simulink model "TorqueControl_QuadRad_MPC"  (R2015b)
settings: Solver=ode4  StartTime=0.0  StopTime=2000  FixedStep=1  RelTol=1e-3
values from neighbouring files (symbols this model uses):
  bicycle = initBicycle(60, 0.01468, 0.79, 0.33, 0.17, 5.5, 24, 50, 48)    [RunSimulinkSim_MPC.m]
  cyclist = initCyclist(0, 30, 183, 75, 80)    [RunSimulinkSim_MPC.m]
  environment = initEnvironment_V2(altitude, distance, fRES, 9.81, 1.2041)    [RunSimulinkSim_MPC.m]
  P_M = P_M_ref+fac.*P_M_ref_exc    [RunSimulinkSim_MPC.m]
  system = initHRmodel(0.0113, 0.0072, 0.0049, 0.0041, 19.8002, 0.0072, cyclist.P_max, cyclist.cadence)    [RunSimulinkSim_MPC.m]
undefined symbols (not defined in the file or in its folder): init, mpc, variation
libraries: simulink x2
settings Model: Creator=Daniel  LastModifiedBy=David
settings DataIOCC: SaveFormat=Array

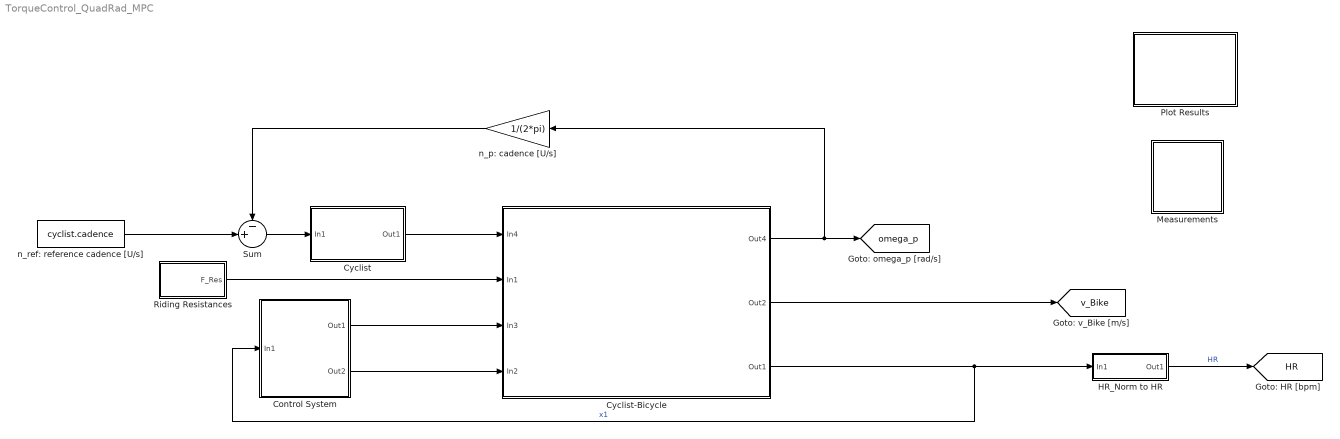
== system TorqueControl_QuadRad_MPC ==
  Control System : Subsystem
  Cyclist : Subsystem
  Cyclist-Bicycle : Subsystem
  HR_Norm to HR : Subsystem
  Measurements : Subsystem
  Plot Results : Subsystem
  Riding Resistances : Subsystem
  Sum : Sum  Inputs=-+|
  n_p: cadence [U/s] : Gain  Gain=1/(2*pi)
  n_ref: reference cadence [U/s] : Constant  Value=cyclist.cadence
  tag scope: HR=global, omega_p=global, v_Bike=global
  wires:
  Cyclist-Bicycle/1(Out4) -> n_p: cadence [U/s]/1, [omega_p]
  n_ref: reference cadence [U/s]/1 -> Sum/2
  n_p: cadence [U/s]/1 -> Sum/1
  Riding Resistances/1(F_Res) -> Cyclist-Bicycle/2(In1)
  Cyclist-Bicycle/2(Out2) -> [v_Bike]
  Cyclist-Bicycle/3(Out1) -> Control System/1(In1), HR_Norm to HR/1(In1)  "x1"
  HR_Norm to HR/1(Out1) -> [HR]  "HR"
  Sum/1 -> Cyclist/1(In1)
  Cyclist/1(Out1) -> Cyclist-Bicycle/1(In4)
  Control System/1(Out1) -> Cyclist-Bicycle/3(In3)
  Control System/2(Out2) -> Cyclist-Bicycle/4(In2)

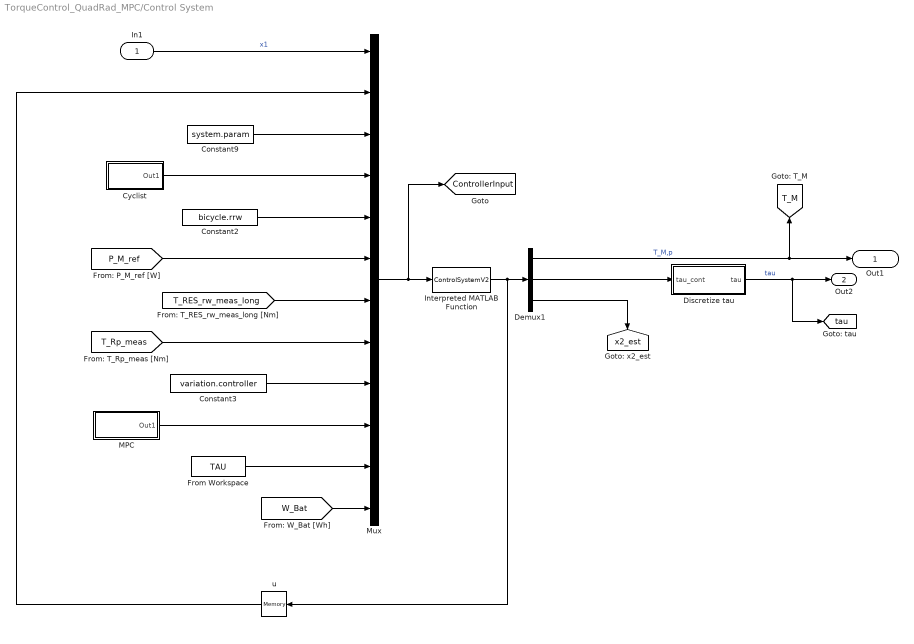
== system TorqueControl_QuadRad_MPC/Control System ==
  In1 : Inport
  Constant2 : Constant  Value=bicycle.rrw
  Constant3 : Constant  Value=variation.controller
  Constant9 : Constant  Value=system.param
  Cyclist : Subsystem
  Demux1 : Demux  Outputs=3
  Discretize tau : MATLAB Function  TreatAsAtomicUnit=on
  From Workspace : FromWorkspace  VariableName=TAU  SampleTime=0
  Interpreted MATLAB Function : MATLABFcn  MATLABFcn=ControlSystemV2  OutputDimensions=3
  MPC : Subsystem
  Mux : Mux  Inputs=12
  u : Memory  X0=[0 init.tau init.x2_est]  InheritSampleTime=on
  Out1 : Outport
  Out2 : Outport  Port=2
  tag scope: ControllerInput=global, T_M=global, tau=global, x2_est=global
  wires:
  In1/1 -> Mux/1  "x1"
  Demux1/3 -> [x2_est]
  Constant2/1 -> Mux/5
  Mux/1 -> [ControllerInput], Interpreted MATLAB Function/1
  Interpreted MATLAB Function/1 -> Demux1/1, u/1
  Constant9/1 -> Mux/3
  [T_RES_rw_meas_long] -> Mux/7
  u/1 -> Mux/2
  [P_M_ref] -> Mux/6
  Demux1/1 -> [T_M], Out1/1  "T_M,p"
  Demux1/2 -> Discretize tau/1(tau_cont)
  Discretize tau/1(tau) -> [tau], Out2/1  "tau"
  Cyclist/1(Out1) -> Mux/4
  [T_Rp_meas] -> Mux/8
  From Workspace/1 -> Mux/11
  Constant3/1 -> Mux/9
  MPC/1(Out1) -> Mux/10
  [W_Bat] -> Mux/12

== system TorqueControl_QuadRad_MPC/Cyclist ==
  In1 : Inport
  T_R,p: Rider torque at pedals [Nm] : simulink/Continuous/PID Controller  Controller=PID  TimeDomain=Discrete-time  SampleTime=-1  IntegratorMethod=Forward Euler  FilterMethod=Forward Euler  Form=Parallel  UseFilter=on  ControllerParametersSource=internal  P=300  I=25  D=0  N=1  InitialConditionSource=internal  InitialConditionForIntegrator=0  InitialConditionForFilter=0  ExternalReset=none  LimitOutput=on  UpperSaturationLimit=1000  LowerSaturationLimit=1  LinearizeAsGain=on  AntiWindupMode=none  Kb=1  TrackingMode=off  Kt=1  PParamMin=[]  PParamMax=[]  IParamMin=[]  IParamMax=[]  DParamMin=[]  DParamMax=[]  NParamMin=[]  NParamMax=[]  KbParamMin=[]  KbParamMax=[]  KtParamMin=[]  KtParamMax=[]  POutMin=[]  POutMax=[]  IOutMin=[]  IOutMax=[]  DOutMin=[]  DOutMax=[]  NOutMin=[]  NOutMax=[]  KbOutMin=[]  KbOutMax=[]  KtOutMin=[]  KtOutMax=[]  IntegratorOutMin=[]  IntegratorOutMax=[]  FilterOutMin=[]  FilterOutMax=[]  SumOutMin=[]  SumOutMax=[]  SumI1OutMin=[]  SumI1OutMax=[]  SumI2OutMin=[]  SumI2OutMax=[]  SumI3OutMin=[]  SumI3OutMax=[]  SumDOutMin=[]  SumDOutMax=[]  SaturationOutMin=[]  SaturationOutMax=[]  IntegratorContinuousStateAttributes=''  IntegratorStateMustResolveToSignalObject=off  IntegratorRTWStateStorageClass=Auto  FilterContinuousStateAttributes=''  FilterStateMustResolveToSignalObject=off  FilterRTWStateStorageClass=Auto  DifferentiatorICPrevScaledInput=0  DifferentiatorOutMin=[]  DifferentiatorOutMax=[]
  Out1 : Outport
  tag scope: T_Rp=global
  wires:
  In1/1 -> T_R,p: Rider torque at pedals [Nm]/1  "e_n"
  T_R,p: Rider torque at pedals [Nm]/1 -> [T_Rp], Out1/1  "T_R,p [Nm]"

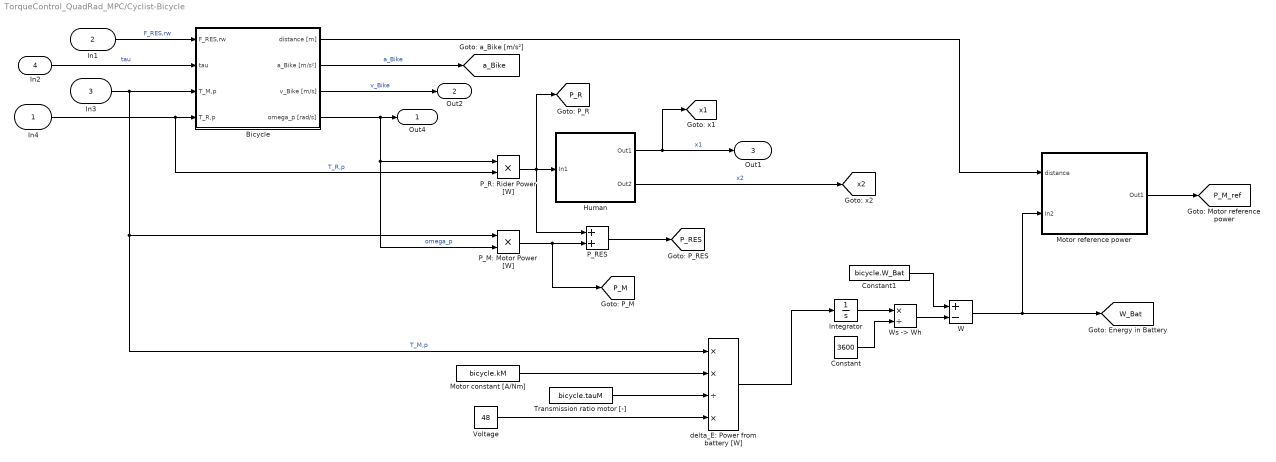
== system TorqueControl_QuadRad_MPC/Cyclist-Bicycle ==
  In4 : Inport
  In1 : Inport  Port=2
  In3 : Inport  Port=3
  In2 : Inport  Port=4
  Bicycle : Subsystem
  Constant : Constant  Value=3600
  Constant1 : Constant  Value=bicycle.W_Bat
  Human : Subsystem
  Integrator : Integrator
  Motor constant [A/Nm] : Constant  Value=bicycle.kM
  Motor reference power : Subsystem
  P_M: Motor Power [W] : Product
  P_R: Rider Power [W] : Product
  P_RES : Sum
  Transmission ratio motor [-] : Constant  Value=bicycle.tauM
  Voltage : Constant  Value=48
  W : Sum  Inputs=+-
  "Ws -> Wh" : Product  Inputs=*/
  delta_E: Power from battery [W] : Product  Inputs=**/*
  Out4 : Outport
  Out2 : Outport  Port=2
  Out1 : Outport  Port=3
  tag scope: P_M=global, P_M_ref=global, P_R=global, P_RES=global, W_Bat=global, a_Bike=global, x1=global, x2=global
  wires:
  P_R: Rider Power [W]/1 -> [P_R], P_RES/1, Human/1(In1)
  Bicycle/3(v_Bike [m/s]) -> Out2/1  "v_Bike"
  Bicycle/2(a_Bike [m/s²]) -> [a_Bike]  "a_Bike"
  Human/2(Out2) -> [x2]  "x2"
  In2/1 -> Bicycle/2(tau)  "tau"
  In3/1 -> P_M: Motor Power [W]/1, delta_E: Power from battery [W]/1, Bicycle/3(T_M,p)  "T_M,p"
  In4/1 -> P_R: Rider Power [W]/2, Bicycle/4(T_R,p)  "T_R,p"
  In1/1 -> Bicycle/1(F_RES,rw)  "F_RES,rw"
  Bicycle/4(omega_p [rad/s]) -> Out4/1, P_M: Motor Power [W]/2, P_R: Rider Power [W]/1  "omega_p"
  Human/1(Out1) -> Out1/1, [x1]  "x1"
  P_M: Motor Power [W]/1 -> [P_M], P_RES/2
  P_RES/1 -> [P_RES]
  Motor constant [A/Nm]/1 -> delta_E: Power from battery [W]/2
  Transmission ratio motor [-]/1 -> delta_E: Power from battery [W]/3
  Voltage/1 -> delta_E: Power from battery [W]/4
  delta_E: Power from battery [W]/1 -> Integrator/1
  Integrator/1 -> "Ws -> Wh"/1
  Constant/1 -> "Ws -> Wh"/2
  "Ws -> Wh"/1 -> W/2
  Constant1/1 -> W/1
  W/1 -> Motor reference power/2(In2), [W_Bat]
  Bicycle/1(distance [m]) -> Motor reference power/1(distance)
  Motor reference power/1(Out1) -> [P_M_ref]

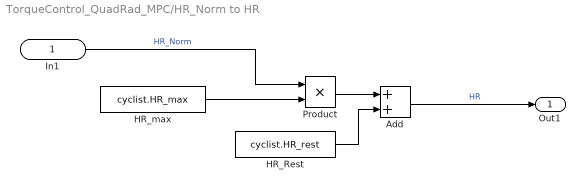
== system TorqueControl_QuadRad_MPC/HR_Norm to HR ==
  In1 : Inport
  Add : Sum
  HR_Rest : Constant  Value=cyclist.HR_rest
  HR_max : Constant  Value=cyclist.HR_max
  Product : Product
  Out1 : Outport
  wires:
  HR_max/1 -> Product/2
  Add/1 -> Out1/1  "HR"
  Product/1 -> Add/1
  HR_Rest/1 -> Add/2
  In1/1 -> Product/1  "HR_Norm"

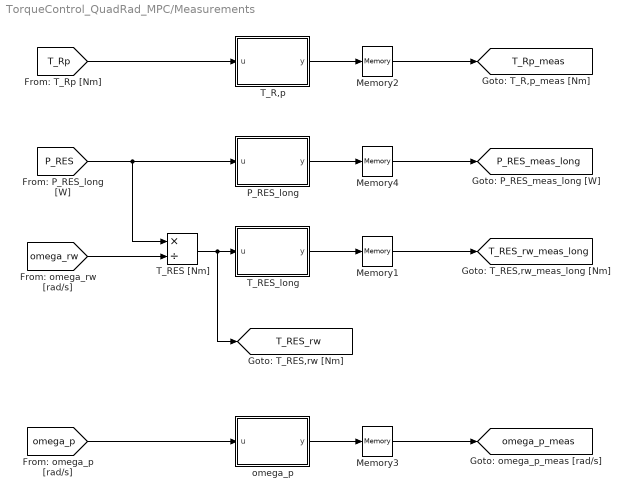
== system TorqueControl_QuadRad_MPC/Measurements ==
  Memory1 : Memory  InheritSampleTime=on
  Memory2 : Memory  InheritSampleTime=on
  Memory3 : Memory  InheritSampleTime=on
  Memory4 : Memory  X0=init.P_RES  InheritSampleTime=on
  P_RES_long : MATLAB Function  TreatAsAtomicUnit=on
  T_R,p : MATLAB Function  TreatAsAtomicUnit=on
  T_RES [Nm] : Product  Inputs=*/
  T_RES_long : MATLAB Function  TreatAsAtomicUnit=on
  omega_p : MATLAB Function  TreatAsAtomicUnit=on
  tag scope: P_RES_meas_long=global, T_RES_rw=global, T_RES_rw_meas_long=global, T_Rp_meas=global, omega_p_meas=global
  wires:
  [P_RES] -> T_RES [Nm]/1, P_RES_long/1(u)
  Memory4/1 -> [P_RES_meas_long]
  P_RES_long/1(y) -> Memory4/1
  [omega_rw] -> T_RES [Nm]/2
  T_RES [Nm]/1 -> [T_RES_rw], T_RES_long/1(u)
  T_RES_long/1(y) -> Memory1/1
  Memory1/1 -> [T_RES_rw_meas_long]
  [T_Rp] -> T_R,p/1(u)
  T_R,p/1(y) -> Memory2/1
  Memory2/1 -> [T_Rp_meas]
  [omega_p] -> omega_p/1(u)
  omega_p/1(y) -> Memory3/1
  Memory3/1 -> [omega_p_meas]

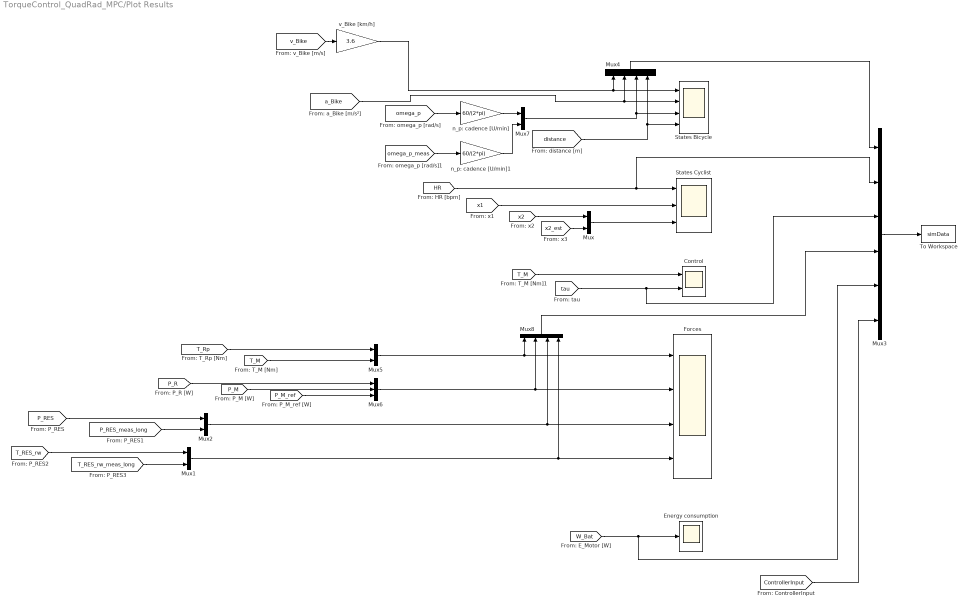
== system TorqueControl_QuadRad_MPC/Plot Results ==
  Control : Scope  NumInputPorts=2
  Energy consumption : Scope
  Forces : Scope  NumInputPorts=4
  Mux{,1..2,5,7} (5 alike) : Mux  Inputs=2
  Mux3 : Mux  Inputs=6
  Mux4 : Mux
  Mux6 : Mux  Inputs=3
  Mux8 : Mux
  States Bicycle : Scope  NumInputPorts=4
  States Cyclist : Scope  NumInputPorts=3
  To Workspace : ToWorkspace  VariableName=simData  SaveFormat=Timeseries  SampleTime=-1
  n_p: cadence [U/min] : Gain  Gain=60/(2*pi)
  n_p: cadence [U/min]1 : Gain  Gain=60/(2*pi)
  v_Bike [km/h] : Gain  Gain=3.6
  wires:
  [omega_p] -> n_p: cadence [U/min]/1
  [v_Bike] -> v_Bike [km/h]/1
  [HR] -> Mux3/2, States Cyclist/1
  [x1] -> States Cyclist/2
  [x2] -> Mux/1
  [P_M] -> Mux6/2
  [P_RES] -> Mux2/1
  [x2_est] -> Mux/2
  Mux/1 -> States Cyclist/3
  [tau] -> Mux3/3, Control/2
  [P_RES_meas_long] -> Mux2/2
  [a_Bike] -> Mux4/2, States Bicycle/2
  [T_Rp] -> Mux5/1
  [P_R] -> Mux6/1
  [distance] -> States Bicycle/4, Mux4/4
  Mux5/1 -> Mux8/1, Forces/1
  Mux6/1 -> Forces/2, Mux8/2
  [T_M] -> Mux5/2
  [T_M] -> Control/1
  Mux2/1 -> Mux8/3, Forces/3
  [T_RES_rw] -> Mux1/1
  [T_RES_rw_meas_long] -> Mux1/2
  Mux1/1 -> Forces/4, Mux8/4
  [P_M_ref] -> Mux6/3
  [W_Bat] -> Mux3/5, Energy consumption/1
  v_Bike [km/h]/1 -> Mux4/1, States Bicycle/1
  Mux3/1 -> To Workspace/1
  Mux4/1 -> Mux3/1
  Mux8/1 -> Mux3/4
  [ControllerInput] -> Mux3/6
  [omega_p_meas] -> n_p: cadence [U/min]1/1
  n_p: cadence [U/min]/1 -> Mux7/1
  n_p: cadence [U/min]1/1 -> Mux7/2
  Mux7/1 -> States Bicycle/3, Mux4/3

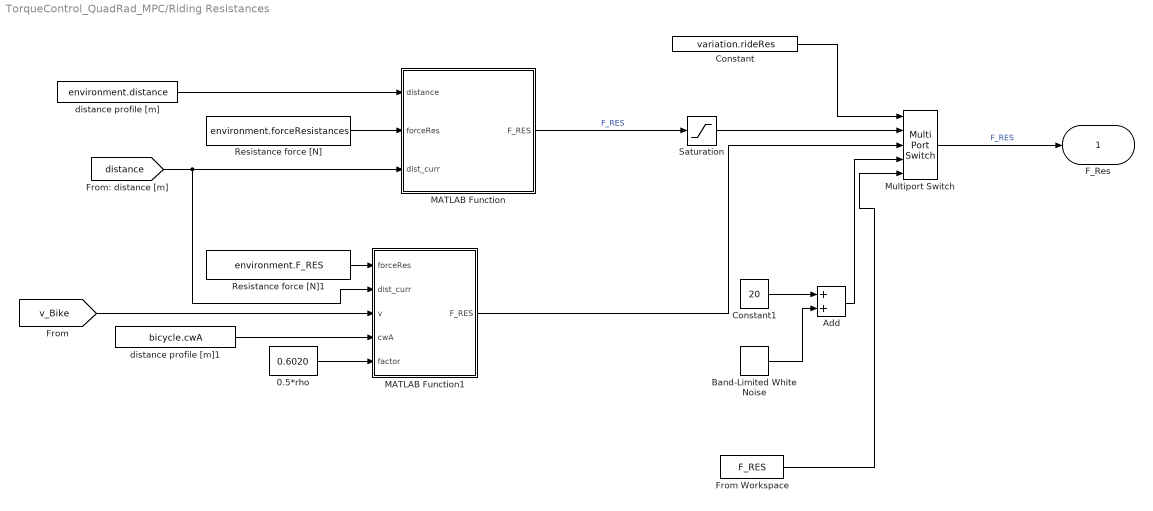
== system TorqueControl_QuadRad_MPC/Riding Resistances ==
  0.5*rho : Constant  Value=0.6020
  Add : Sum
  Band-Limited White Noise : simulink/Sources/Band-Limited White Noise  Cov=[10]  Ts=1  seed=[23341]
  Constant : Constant  Value=variation.rideRes
  Constant1 : Constant  Value=20
  From Workspace : FromWorkspace  VariableName=F_RES  SampleTime=0
  MATLAB Function : MATLAB Function  TreatAsAtomicUnit=on
  MATLAB Function1 : MATLAB Function  TreatAsAtomicUnit=on
  Multiport Switch : MultiPortSwitch  Inputs=4
  Resistance force [N] : Constant  Value=environment.forceResistances
  Resistance force [N]1 : Constant  Value=environment.F_RES
  Saturation : Saturate  UpperLimit=150  LowerLimit=0
  distance profile [m] : Constant  Value=environment.distance
  distance profile [m]1 : Constant  Value=bicycle.cwA
  F_Res : Outport
  wires:
  [distance] -> MATLAB Function/3(dist_curr), MATLAB Function1/2(dist_curr)
  Multiport Switch/1 -> F_Res/1  "F_RES"
  distance profile [m]/1 -> MATLAB Function/1(distance)
  Resistance force [N]/1 -> MATLAB Function/2(forceRes)
  Constant/1 -> Multiport Switch/1
  MATLAB Function/1(F_RES) -> Saturation/1  "F_RES"
  Constant1/1 -> Add/1
  Band-Limited White Noise/1 -> Add/2
  Add/1 -> Multiport Switch/4
  From Workspace/1 -> Multiport Switch/5
  Saturation/1 -> Multiport Switch/2
  [v_Bike] -> MATLAB Function1/3(v)
  distance profile [m]1/1 -> MATLAB Function1/4(cwA)
  0.5*rho/1 -> MATLAB Function1/5(factor)
  Resistance force [N]1/1 -> MATLAB Function1/1(forceRes)
  MATLAB Function1/1(F_RES) -> Multiport Switch/3

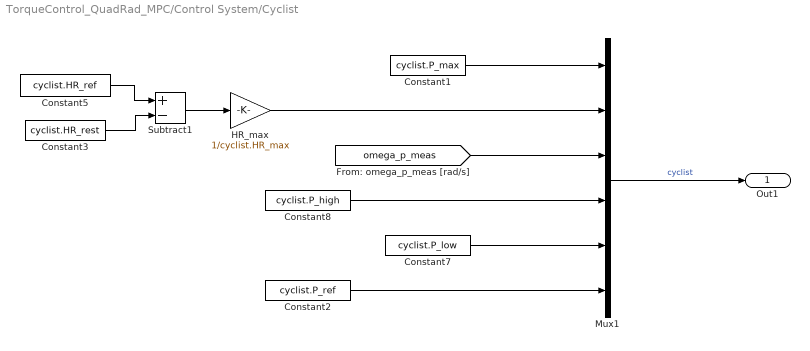
== system TorqueControl_QuadRad_MPC/Control System/Cyclist ==
  Constant1 : Constant  Value=cyclist.P_max
  Constant2 : Constant  Value=cyclist.P_ref
  Constant3 : Constant  Value=cyclist.HR_rest
  Constant5 : Constant  Value=cyclist.HR_ref
  Constant7 : Constant  Value=cyclist.P_low
  Constant8 : Constant  Value=cyclist.P_high
  HR_max : Gain  Gain=1/cyclist.HR_max
  Mux1 : Mux  Inputs=6
  Subtract1 : Sum  Inputs=+-
  Out1 : Outport
  wires:
  HR_max/1 -> Mux1/2
  [omega_p_meas] -> Mux1/3
  Mux1/1 -> Out1/1  "cyclist"
  Constant1/1 -> Mux1/1
  Constant3/1 -> Subtract1/2
  Constant5/1 -> Subtract1/1
  Subtract1/1 -> HR_max/1
  Constant8/1 -> Mux1/4
  Constant7/1 -> Mux1/5
  Constant2/1 -> Mux1/6

== system TorqueControl_QuadRad_MPC/Control System/MPC ==
  Constant1 : Constant  Value=mpc.weights
  Constant2 : Constant  Value=mpc.predHor
  Mux : Mux  Inputs=2
  Out1 : Outport
  wires:
  Constant1/1 -> Mux/1
  Mux/1 -> Out1/1  "mpc"
  Constant2/1 -> Mux/2

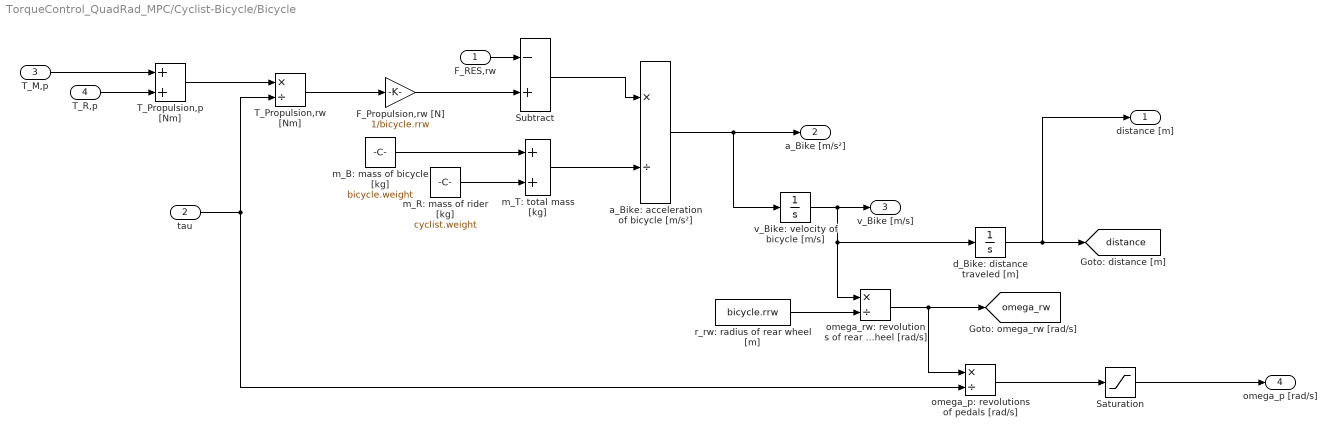
== system TorqueControl_QuadRad_MPC/Cyclist-Bicycle/Bicycle ==
  F_RES,rw : Inport
  tau : Inport  Port=2
  T_M,p : Inport  Port=3
  T_R,p : Inport  Port=4
  F_Propulsion,rw [N] : Gain  Gain=1/bicycle.rrw
  Saturation : Saturate  UpperLimit=1000  LowerLimit=0
  Subtract : Sum  Inputs=-+
  T_Propulsion,p [Nm] : Sum
  T_Propulsion,rw [Nm] : Product  Inputs=*/
  a_Bike: acceleration of bicycle [m/s²] : Product  Inputs=*/
  d_Bike: distance traveled [m] : Integrator  InitialCondition=init.d_Bike
  m_B: mass of bicycle [kg] : Constant  Value=bicycle.weight
  m_R: mass of rider [kg] : Constant  Value=cyclist.weight
  m_T: total mass [kg] : Sum
  omega_p: revolutions of pedals [rad/s] : Product  Inputs=*/
  omega_rw: revolutions of rear wheel [rad/s] : Product  Inputs=*/
  r_rw: radius of rear wheel [m] : Constant  Value=bicycle.rrw
  v_Bike: velocity of bicycle [m/s] : Integrator  InitialCondition=init.v_Bike
  distance [m] : Outport
  a_Bike [m/s²] : Outport  Port=2
  v_Bike [m/s] : Outport  Port=3
  omega_p [rad/s] : Outport  Port=4
  tag scope: distance=global, omega_rw=global
  wires:
  m_B: mass of bicycle [kg]/1 -> m_T: total mass [kg]/1
  T_R,p/1 -> T_Propulsion,p [Nm]/2
  a_Bike: acceleration of bicycle [m/s²]/1 -> a_Bike [m/s²]/1, v_Bike: velocity of bicycle [m/s]/1
  m_T: total mass [kg]/1 -> a_Bike: acceleration of bicycle [m/s²]/2
  m_R: mass of rider [kg]/1 -> m_T: total mass [kg]/2
  T_M,p/1 -> T_Propulsion,p [Nm]/1
  F_RES,rw/1 -> Subtract/1
  tau/1 -> T_Propulsion,rw [Nm]/2, omega_p: revolutions of pedals [rad/s]/2
  Subtract/1 -> a_Bike: acceleration of bicycle [m/s²]/1
  r_rw: radius of rear wheel [m]/1 -> omega_rw: revolutions of rear wheel [rad/s]/2
  v_Bike: velocity of bicycle [m/s]/1 -> omega_rw: revolutions of rear wheel [rad/s]/1, d_Bike: distance traveled [m]/1, v_Bike [m/s]/1
  omega_rw: revolutions of rear wheel [rad/s]/1 -> [omega_rw], omega_p: revolutions of pedals [rad/s]/1
  omega_p: revolutions of pedals [rad/s]/1 -> Saturation/1
  T_Propulsion,rw [Nm]/1 -> F_Propulsion,rw [N]/1
  d_Bike: distance traveled [m]/1 -> distance [m]/1, [distance]
  T_Propulsion,p [Nm]/1 -> T_Propulsion,rw [Nm]/1
  F_Propulsion,rw [N]/1 -> Subtract/2
  Saturation/1 -> omega_p [rad/s]/1

== system TorqueControl_QuadRad_MPC/Cyclist-Bicycle/Human ==
  In1 : Inport
  Nonlinear Human Model : Subsystem
  Power to Power_Norm : Subsystem
  Out1 : Outport
  Out2 : Outport  Port=2
  wires:
  In1/1 -> Power to Power_Norm/1(In1)  "P_Rider"
  Nonlinear Human Model/1(Out1) -> Out1/1  "x1"
  Nonlinear Human Model/2(Out2) -> Out2/1  "x2"
  Power to Power_Norm/1(Out1) -> Nonlinear Human Model/1(In1)

== system TorqueControl_QuadRad_MPC/Cyclist-Bicycle/Motor reference power ==
  distance : Inport
  In2 : Inport  Port=2
  Constant : Constant  Value=variation.tripInfo
  Constant1 : Constant  Value=250
  Trip Optimization : Subsystem
  Out1 : Outport
  wires:
  Trip Optimization/1(Out1) -> Out1/1  "P_M_ref"
  distance/1 -> Trip Optimization/1(distance)  "distance"
  In2/1 -> Trip Optimization/2(In2)  "W_Bat"
  Constant1/1 -> Trip Optimization/3(distance1)
  Constant/1 -> Trip Optimization/4(distance3)

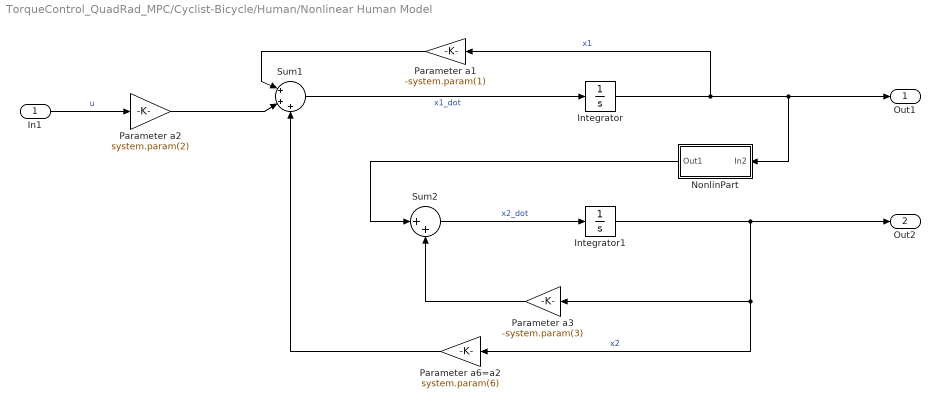
== system TorqueControl_QuadRad_MPC/Cyclist-Bicycle/Human/Nonlinear Human Model ==
  In1 : Inport
  Integrator : Integrator  InitialCondition=init.x1
  Integrator1 : Integrator  InitialCondition=init.x2
  NonlinPart : Subsystem
  Parameter a1 : Gain  Gain=-system.param(1)
  Parameter a2 : Gain  Gain=system.param(2)
  Parameter a3 : Gain  Gain=-system.param(3)
  Parameter a6=a2 : Gain  Gain=system.param(6)
  Sum1 : Sum  Inputs=|+++
  Sum2 : Sum  Inputs=|++
  Out1 : Outport
  Out2 : Outport  Port=2
  wires:
  Integrator/1 -> Parameter a1/1, Out1/1, NonlinPart/1(In2)  "x1"
  Integrator1/1 -> Parameter a6=a2/1, Parameter a3/1, Out2/1  "x2"
  Parameter a6=a2/1 -> Sum1/3
  NonlinPart/1(Out1) -> Sum2/1
  Sum2/1 -> Integrator1/1  "x2_dot"
  Parameter a3/1 -> Sum2/2
  Parameter a1/1 -> Sum1/1
  In1/1 -> Parameter a2/1  "u"
  Sum1/1 -> Integrator/1  "x1_dot"
  Parameter a2/1 -> Sum1/2

== system TorqueControl_QuadRad_MPC/Cyclist-Bicycle/Human/Power to Power_Norm ==
  In1 : Inport
  Constant : Constant  Value=cyclist.P_max
  Divide : Product  Inputs=*/
  Saturation : Saturate  UpperLimit=cyclist.P_max  LowerLimit=0  ZeroCross=off
  Out1 : Outport
  wires:
  Constant/1 -> Divide/2
  Divide/1 -> Out1/1  "Power_Norm"
  In1/1 -> Saturation/1  "Power"
  Saturation/1 -> Divide/1

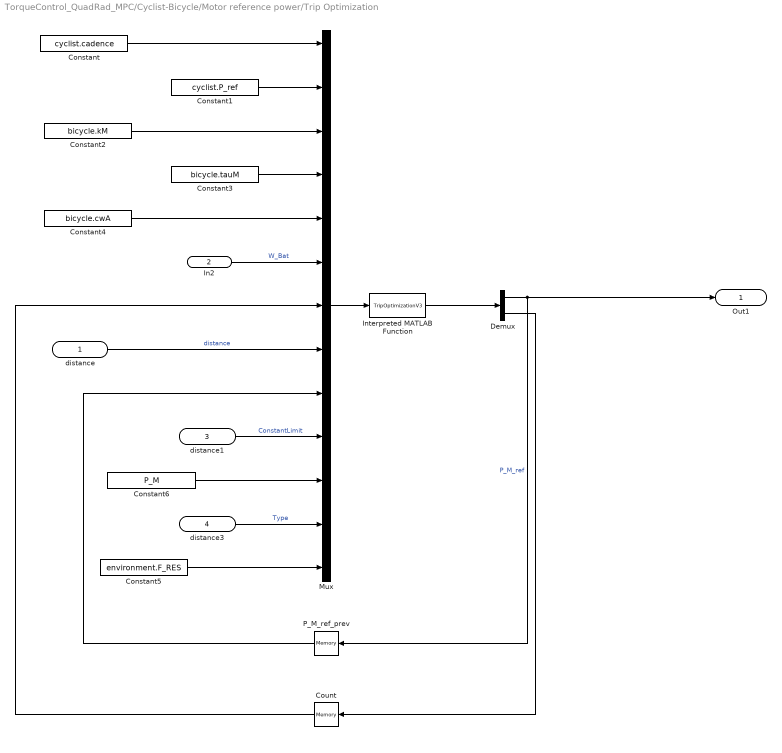
== system TorqueControl_QuadRad_MPC/Cyclist-Bicycle/Motor reference power/Trip Optimization ==
  distance : Inport
  In2 : Inport  Port=2
  distance1 : Inport  Port=3
  distance3 : Inport  Port=4
  Constant : Constant  Value=cyclist.cadence
  Constant1 : Constant  Value=cyclist.P_ref
  Constant2 : Constant  Value=bicycle.kM
  Constant3 : Constant  Value=bicycle.tauM
  Constant4 : Constant  Value=bicycle.cwA
  Constant5 : Constant  Value=environment.F_RES
  Constant6 : Constant  Value=P_M
  Count : Memory
  Demux : Demux  Outputs=2
  Interpreted MATLAB Function : MATLABFcn  MATLABFcn=TripOptimizationV3  OutputDimensions=2
  Mux : Mux  Inputs=13
  P_M_ref_prev : Memory
  Out1 : Outport
  wires:
  Count/1 -> Mux/7
  Constant/1 -> Mux/1
  Constant1/1 -> Mux/2
  Constant2/1 -> Mux/3
  Constant3/1 -> Mux/4
  P_M_ref_prev/1 -> Mux/9
  Interpreted MATLAB Function/1 -> Demux/1
  In2/1 -> Mux/6  "W_Bat"
  Constant4/1 -> Mux/5
  Mux/1 -> Interpreted MATLAB Function/1
  Demux/2 -> Count/1
  Demux/1 -> P_M_ref_prev/1, Out1/1  "P_M_ref"
  distance/1 -> Mux/8  "distance"
  Constant5/1 -> Mux/13
  distance1/1 -> Mux/10  "ConstantLimit"
  distance3/1 -> Mux/12  "Type"
  Constant6/1 -> Mux/11

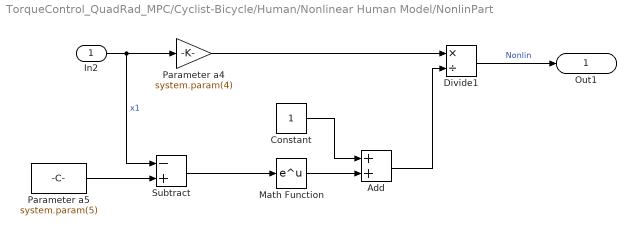
== system TorqueControl_QuadRad_MPC/Cyclist-Bicycle/Human/Nonlinear Human Model/NonlinPart ==
  In2 : Inport
  Add : Sum
  Constant : Constant
  Divide1 : Product  Inputs=*/
  Math Function : Math  SaturateOnIntegerOverflow=on
  Parameter a4 : Gain  Gain=system.param(4)
  Parameter a5 : Constant  Value=system.param(5)
  Subtract : Sum  Inputs=-+
  Out1 : Outport
  wires:
  Parameter a4/1 -> Divide1/1
  In2/1 -> Subtract/1, Parameter a4/1  "x1"
  Divide1/1 -> Out1/1  "Nonlin"
  Constant/1 -> Add/1
  Parameter a5/1 -> Subtract/2
  Math Function/1 -> Add/2
  Add/1 -> Divide1/2
  Subtract/1 -> Math Function/1

== matlab function TorqueControl_QuadRad_MPC/Control System/Discretize tau ==
  data: tau_cont input; tau output
function tau = fcn(tau_cont)
%#codegen

type = 2;

if type==1
    if tau_cont>2.3
        tau = 2.5;
    elseif tau_cont>2.0
        tau = 2.1;
    elseif tau_cont>1.8
        tau = 1.9;
    elseif tau_cont>1.6
        tau = 1.7;
    elseif tau_cont>1.4
        tau = 1.5;
    elseif tau_cont>1.2
        tau = 1.3;
    else
        tau = 1.1;
    end
else
    tau = tau_cont;
end

== matlab function TorqueControl_QuadRad_MPC/Measurements/T_RES_long ==
  data: u input; y output
function y = fcn(u)
%#codegen
persistent i buf bufSum;
span = 60;
if isempty(buf)
    buf = zeros(1,span);
    bufSum = 0;
    i = 0;
end

j = mod(i,span);

bufSum = bufSum - buf(j+1);
buf(j+1) = u;
bufSum = bufSum + u;
i = i + 1;
if i < span
    y = bufSum/(i+1);
else
    y = bufSum/span;
end

== matlab function TorqueControl_QuadRad_MPC/Measurements/T_R,p ==
  data: u input; y output
function y = fcn(u)
%#codegen
persistent i buf bufSum;
span = 2;
if isempty(buf)
    buf = zeros(1,span);
    bufSum = 0;
    i = 0;
end

j = mod(i,span);

bufSum = bufSum - buf(j+1);
buf(j+1) = u;
bufSum = bufSum + u;
i = i + 1;
if i < span
    y = bufSum/(i+1);
else
    y = bufSum/span;
end

== matlab function TorqueControl_QuadRad_MPC/Measurements/P_RES_long ==
  data: u input; y output
function y = fcn(u)
%#codegen
persistent i buf bufSum;
span = 60;
if isempty(buf)
    buf = zeros(1,span);
    bufSum = 0;
    i = 0;
end

j = mod(i,span);

bufSum = bufSum - buf(j+1);
buf(j+1) = u;
bufSum = bufSum + u;
i = i + 1;
if i < span
    y = bufSum/(i+1);
else
    y = bufSum/span;
end

== matlab function TorqueControl_QuadRad_MPC/Measurements/omega_p ==
  data: u input; y output
function y = fcn(u)
%#codegen
persistent i buf bufSum;
span = 20;
if isempty(buf)
    buf = zeros(1,span);
    bufSum = 0;
    i = 0;
end

j = mod(i,span);

bufSum = bufSum - buf(j+1);
buf(j+1) = u;
bufSum = bufSum + u;
i = i + 1;
if i < span
    y = bufSum/(i+1);
else
    y = bufSum/span;
end

== matlab function TorqueControl_QuadRad_MPC/Riding Resistances/MATLAB Function1 ==
  data: forceRes input; F_RES output; dist_curr input; v input; cwA input; factor input
function F_RES = fcn(forceRes, dist_curr, v, cwA, factor)
%#codegen

currentSection = round(round(dist_curr)/500)+1;

if currentSection>20
    currentSection=20;
end

f_RES = forceRes(currentSection);

F_air = factor*cwA*v^3;

F_RES = F_air + f_RES;

== matlab function TorqueControl_QuadRad_MPC/Riding Resistances/MATLAB Function ==
  data: distance input; forceRes input; dist_curr input; F_RES output
function F_RES = fcn(distance, forceRes, dist_curr)
%#codegen

d_curr = mod(round(dist_curr),9970);

f_RES = interp1(distance,forceRes,(0:1:9970)');

F_RES = f_RES(d_curr+1,1);
